simulink model "opcional_5"  (R2018b)
settings: Solver=VariableStepAuto  StartTime=0  StopTime=8  RelTol=1e-3
libraries: dspsrcs4 x3, simulink x1
settings Model: Creator=carta  LastModifiedBy=carta

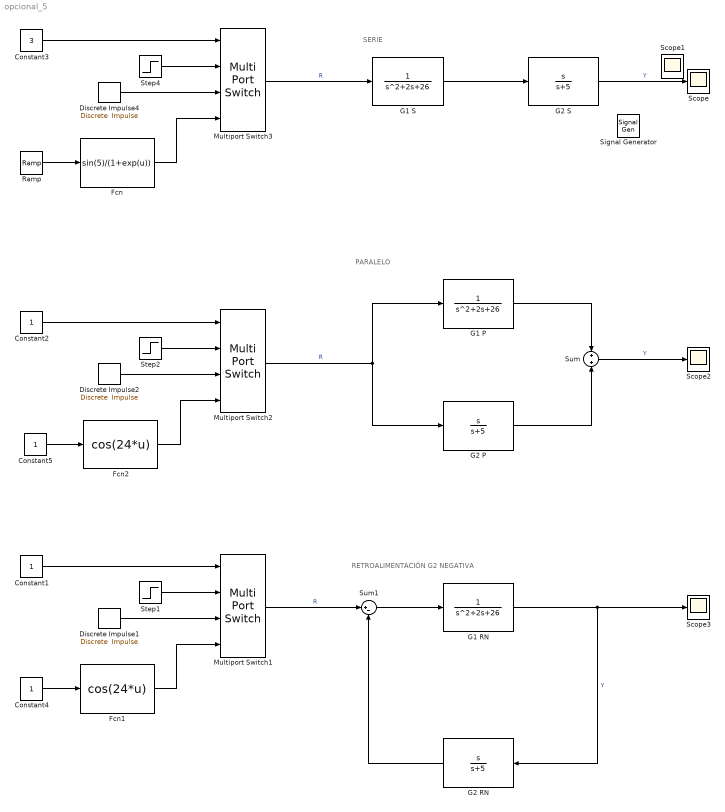
== system opcional_5 ==
  note: RETROALIMENTACIÓN G2 NEGATIVA
  note: PARALELO
  note: SERIE
  Constant{1..2,4..5} (4 alike) : Constant
  Constant3 : Constant  Value=3
  Discrete Impulse1 : dspsrcs4/Discrete  Impulse  Delay=0  SampleTime=0.1  FrameSample=1  OutputFrames=off  dataType=double  isSigned=on  wordLen=16  udDataType=sfix(16)  fracBitsMode=Best precision  numFracBits=15  OutDataTypeStr=double  LastOutDataTypeStr=double
  Discrete Impulse2 : dspsrcs4/Discrete  Impulse  Delay=0  SampleTime=0.1  FrameSample=1  OutputFrames=off  dataType=double  isSigned=on  wordLen=16  udDataType=sfix(16)  fracBitsMode=Best precision  numFracBits=15  OutDataTypeStr=double  LastOutDataTypeStr=double
  Discrete Impulse4 : dspsrcs4/Discrete  Impulse  Delay=0  SampleTime=0.1  FrameSample=1  OutputFrames=off  dataType=double  isSigned=on  wordLen=16  udDataType=sfix(16)  fracBitsMode=Best precision  numFracBits=15  OutDataTypeStr=double  LastOutDataTypeStr=double
  Fcn : Fcn  Expr=sin(5)/(1+exp(u))
  Fcn1 : Fcn  Expr=cos(24*u)
  Fcn2 : Fcn  Expr=cos(24*u)
  G1 P : TransferFcn  Denominator=[1 2 26]
  G1 RN : TransferFcn  Denominator=[1 2 26]
  G1 S : TransferFcn  Denominator=[1 2 26]
  G2 P : TransferFcn  Numerator=[1 0]  Denominator=[1 5]
  G2 RN : TransferFcn  Numerator=[1 0]  Denominator=[1 5]
  G2 S : TransferFcn  Numerator=[1 0]  Denominator=[1 5]
  Multiport Switch1 : MultiPortSwitch  DataPortOrder=Specify indices
  Multiport Switch2 : MultiPortSwitch  DataPortOrder=Specify indices
  Multiport Switch3 : MultiPortSwitch  DataPortOrder=Specify indices
  Ramp : simulink/Sources/Ramp  slope=1  start=0  InitialOutput=0
  Scope{,1..3} (4 alike) : Scope
  Step1 : Step  Time=0  SampleTime=0
  Step2 : Step  Time=0  SampleTime=0
  Step4 : Step  Time=0  SampleTime=0
  Sum : Sum  Inputs=+|+
  Sum1 : Sum  Inputs=|+-
  Signal Generator : SignalGenerator  IOType=siggen
  wires:
  G2 S/1 -> Scope/1  "Y"
  G1 S/1 -> G2 S/1
  Multiport Switch3/1 -> G1 S/1  "R"
  G1 P/1 -> Sum/1
  G2 P/1 -> Sum/2
  Multiport Switch2/1 -> G1 P/1, G2 P/1  "R"
  Sum/1 -> Scope2/1  "Y"
  G1 RN/1 -> G2 RN/1, Scope3/1  "Y"
  G2 RN/1 -> Sum1/2
  Multiport Switch1/1 -> Sum1/1  "R"
  Sum1/1 -> G1 RN/1
  Step1/1 -> Multiport Switch1/2
  Constant1/1 -> Multiport Switch1/1
  Discrete Impulse1/1 -> Multiport Switch1/3
  Step2/1 -> Multiport Switch2/2
  Constant2/1 -> Multiport Switch2/1
  Discrete Impulse2/1 -> Multiport Switch2/3
  Step4/1 -> Multiport Switch3/2
  Constant3/1 -> Multiport Switch3/1
  Discrete Impulse4/1 -> Multiport Switch3/3
  Fcn/1 -> Multiport Switch3/4
  Ramp/1 -> Fcn/1
  Constant4/1 -> Fcn1/1
  Fcn1/1 -> Multiport Switch1/4
  Constant5/1 -> Fcn2/1
  Fcn2/1 -> Multiport Switch2/4
